simulink model "pruebaswitch"  (R2016b)
settings: Solver=VariableStepAuto  StartTime=0.0  StopTime=10.0  RelTol=1e-3
undefined symbols (not defined in the file): LD
settings Model: Creator=Uxío  LastModifiedBy=Uxío

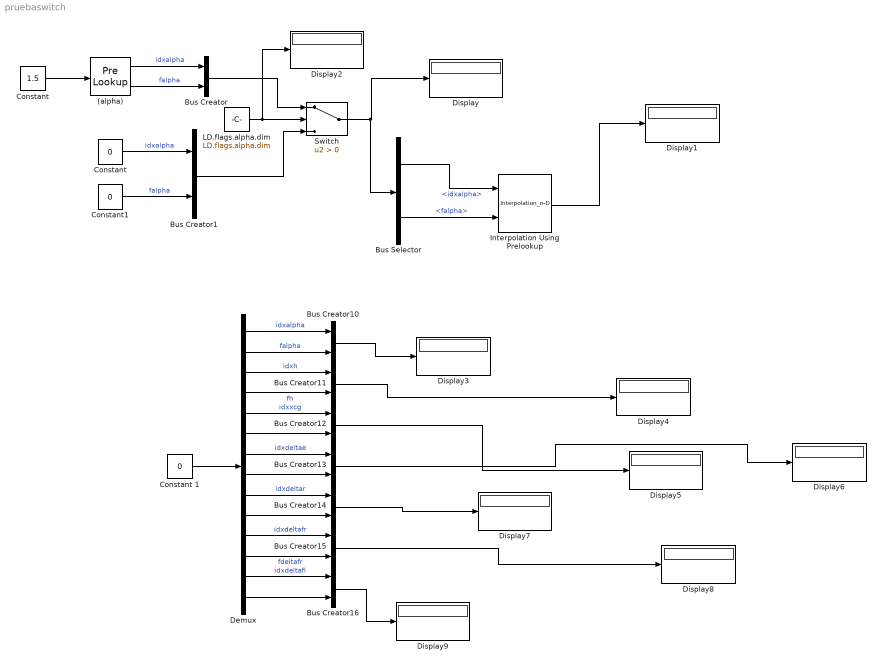
== system pruebaswitch ==
  (alpha) : PreLookup  BreakpointsData=LD.alpha  BeginIndexSearchUsingPreviousIndexResult=on  DiagnosticForOutOfRangeInput=Warning  IndexDataTypeStr=int32  FractionDataTypeStr=double
  Bus Creator{,1,10..16} (9 alike) : BusCreator  Inputs=2
  Bus Selector : BusSelector  OutputSignals=idxalpha,falpha
  Constant : Constant  Value=1.5
  "Constant " : Constant  Value=0
  Constant 1 : Constant  Value=0
  Constant1 : Constant  Value=0
  Demux : Demux  Outputs=14
  Display{,1..9} (10 alike) : Display
  Interpolation Using Prelookup : Interpolation_n-D  NumberOfTableDimensions=1  Table=[10,20]  InternalRulePriority=Speed
      settings: InputPortMap=u0,u1
  LD.flags.alpha.dim : Constant  Value=LD.flags.alpha.dim
  Switch : Switch  Criteria=u2 > Threshold
  wires:
  (alpha)/2 -> Bus Creator/2  "falpha"
  Switch/1 -> Bus Selector/1, Display/1
  LD.flags.alpha.dim/1 -> Display2/1, Switch/2
  (alpha)/1 -> Bus Creator/1  "idxalpha"
  Constant/1 -> (alpha)/1
  "Constant "/1 -> Bus Creator1/1  "idxalpha"
  Constant1/1 -> Bus Creator1/2  "falpha"
  Bus Creator/1 -> Switch/1
  Bus Creator1/1 -> Switch/3
  Bus Selector/1 -> Interpolation Using Prelookup/1  "<idxalpha>"
  Bus Selector/2 -> Interpolation Using Prelookup/2  "<falpha>"
  Interpolation Using Prelookup/1 -> Display1/1
  Demux/2 -> Bus Creator10/2  "falpha"
  Demux/1 -> Bus Creator10/1  "idxalpha"
  Demux/4 -> Bus Creator11/2  "fh"
  Demux/3 -> Bus Creator11/1  "idxh"
  Demux/5 -> Bus Creator12/1  "idxxcg"
  Demux/6 -> Bus Creator12/2
  Demux/8 -> Bus Creator13/2
  Demux/7 -> Bus Creator13/1  "idxdeltae"
  Demux/10 -> Bus Creator14/2
  Demux/9 -> Bus Creator14/1  "idxdeltar"
  Demux/12 -> Bus Creator15/2  "fdeltafr"
  Demux/11 -> Bus Creator15/1  "idxdeltafr"
  Demux/13 -> Bus Creator16/1  "idxdeltafl"
  Demux/14 -> Bus Creator16/2
  Constant 1/1 -> Demux/1
  Bus Creator10/1 -> Display3/1
  Bus Creator11/1 -> Display4/1
  Bus Creator12/1 -> Display5/1
  Bus Creator13/1 -> Display6/1
  Bus Creator14/1 -> Display7/1
  Bus Creator15/1 -> Display8/1
  Bus Creator16/1 -> Display9/1
